simulink model "state_space_all_reduce_uio"  (R2018a)
settings: Solver=FixedStepAuto  StartTime=0.0  StopTime=3  FixedStep=tm  MaxStep=1e-4  RelTol=1e-5  AbsTol=1e-5
InitFcn:
  | SimulinkInit_linea_transmision
values from neighbouring files (symbols this model uses):
  b = 4.91    [SimulinkInit_linea_transmision.m]
  C = 1    [SimulinkInit_linea_transmision.m]
  C1 = 22e-6    (= 2.2e-05)    [SimulinkInit_linea_transmision.m]
  C2 = 22e-6    (= 2.2e-05)    [SimulinkInit_linea_transmision.m]
  C3 = 610e-6    (= 0.00061)    [SimulinkInit_linea_transmision.m]
  Cl = 20000e-6    (= 0.02)    [SimulinkInit_linea_transmision.m]
  Jd = 0.3    [SimulinkInit_linea_transmision.m]
  K = 25    [SimulinkInit_linea_transmision.m]    (also in uio_linear.m = K1+E*H)
  K1 = 9.66    [SimulinkInit_linea_transmision.m]    (also in uio_linear.m = K1')
  K11 = 0.8    [SimulinkInit_linea_transmision.m]
  K1d = 1.15    [SimulinkInit_linea_transmision.m]
  K2 = 6.97    [SimulinkInit_linea_transmision.m]
  K22 = 0.2    [SimulinkInit_linea_transmision.m]
  K2d = 1    [SimulinkInit_linea_transmision.m]
  K3 = 31.8    [SimulinkInit_linea_transmision.m]
  K33 = 0.23    [SimulinkInit_linea_transmision.m]
  K3d = 1    [SimulinkInit_linea_transmision.m]
  K4 = 15.1    [SimulinkInit_linea_transmision.m]
  Kd = 0.02    [SimulinkInit_linea_transmision.m]
  Kdc = 0.02    [SimulinkInit_linea_transmision.m]
  Kf = 1    [SimulinkInit_linea_transmision.m]
  Kh = 1.2    [SimulinkInit_linea_transmision.m]
  Ks = 21.5    [SimulinkInit_linea_transmision.m]
  Ksc = 3    [SimulinkInit_linea_transmision.m]
  Kv = 1    [SimulinkInit_linea_transmision.m]
  L = 5.2    [SimulinkInit_linea_transmision.m]
  L1 = 40e-3    (= 0.04)    [SimulinkInit_linea_transmision.m]
  L2 = 30e-3    (= 0.03)    [SimulinkInit_linea_transmision.m]
  L3 = 5e-3    (= 0.005)    [SimulinkInit_linea_transmision.m]
  L4 = 35e-6    (= 3.5e-05)    [SimulinkInit_linea_transmision.m]
  L5 = 22e-6    (= 2.2e-05)    [SimulinkInit_linea_transmision.m]
  L6 = 10e-6    (= 1e-05)    [SimulinkInit_linea_transmision.m]
  Pd = 0.1    [SimulinkInit_linea_transmision.m]
  R = 10    [SimulinkInit_linea_transmision.m]
  R1 = 0.1    [SimulinkInit_linea_transmision.m]
  R2 = 0.2    [SimulinkInit_linea_transmision.m]
  R3 = 1e-3    (= 0.001)    [SimulinkInit_linea_transmision.m]
  R4 = 0.005    [SimulinkInit_linea_transmision.m]
  R5 = 0.0012    [SimulinkInit_linea_transmision.m]
  R6 = 0.001    [SimulinkInit_linea_transmision.m]
  RL = 10    [SimulinkInit_linea_transmision.m]
  Sbin = 13.8    [SimulinkInit_linea_transmision.m]
  Svin = 2.91    [SimulinkInit_linea_transmision.m]
  T1 = 0.4    [SimulinkInit_linea_transmision.m]
  T2 = 1    [SimulinkInit_linea_transmision.m]
  T3 = 15    [SimulinkInit_linea_transmision.m]
  T4 = 2.5    [SimulinkInit_linea_transmision.m]
  Tao1d = 0.5    [SimulinkInit_linea_transmision.m]
  Tao2d = 0.125    [SimulinkInit_linea_transmision.m]
  Tcd = 0.2    [SimulinkInit_linea_transmision.m]
  Tcr = 0.01    [SimulinkInit_linea_transmision.m]
  Tf = 0.04    [SimulinkInit_linea_transmision.m]
  Tr = 950    [SimulinkInit_linea_transmision.m]
  Tt = 450    [SimulinkInit_linea_transmision.m]
  Ttd = 0.04    [SimulinkInit_linea_transmision.m]
  Tv = 0.05    [SimulinkInit_linea_transmision.m]
  V = 20    [SimulinkInit_linea_transmision.m]
  wref = 70000    [SimulinkInit_linea_transmision.m]
  X_acid = 1.2    [SimulinkInit_linea_transmision.m]
  X_meth = 0.35    [SimulinkInit_linea_transmision.m]
  Z = 3    [SimulinkInit_linea_transmision.m]
undefined symbols (not defined in the file or in its folder): Ad, ataque, Bd, c11, c12, c13, c14, C1o, c21, c22, c23, c24, C2o, c31, c32, c33, c34, C3o, c41, c42, c43, c44, C4o, Cd, F1, F2, F3, F4, H1, H2, H3, H4, K1U, K2U, K3U, K4U, T1s, T2s, T3s, T4s, T5s, tao1, tao2, taod, tm, uio1r, uio2r, uio3r, uio4r
libraries: neural x277, dsparch4 x4, powerlib_meascontrol x4, mpclib x1, simulink x1
(part 16 of 16)

== matlab function state_space_all_reduce_uio/LinearProg3 ==
  data: Q_load input; Qbo output; Q_e_alt input; kb input; kd input; QdMax input; QbMax input; Qdo output; Q_e_alt_min input
function [Qbo, Qdo] = fcn(Q_load, Q_e_alt, kb, kd, QdMax, QbMax, Q_e_alt_min)

% Q_load es la Qotencia que se requiere en la carga.

% Q_e_alt es la Qotencia estimada de generacion de las energias
% alternativas

% kb y kd son los Qesos de las funcion de costo.

% las salidas son las Qotencias oQtimas Qara bio y diesel

Qb=0;
Qd=0;

D_Q_e_alt = Q_e_alt - Q_e_alt_min; % suQeraavit de energia alternativa.

flagDelt = 0;

if(D_Q_e_alt >= Q_load)
    flagDelt = 1;
end
   

if(flagDelt==0)
    Q_trad = Q_load - D_Q_e_alt;
    % flag: variable que indica si tiene sentido evaluar los
    % if's que se encuentran mas adelante. es decir, si flag = 0 
    % desQues del Qrimer if entonces NO se le esta Qidiendo al sistema
    % mas Qotencia de la que Quede generar y Qortanto el Qroblema de 
    % oQtimizacion lineal tiene sentido.
    % entonces 
    flag=0;

    if(Q_trad>QdMax+QbMax)
        Qd=QdMax;
        Qb=QbMax;
        flag=1;
    end

    % si ambas energias tienen el mismo factor de costo.
    if(kd==kb && flag==0)
        Qb=Q_trad/2;
        Qd=Q_trad/2;
    end

    % si la energia diesel es mas cara que la biomasa.
    if(kd>kb && flag==0)
        if(Q_trad<=QbMax)
            Qb=Q_trad;
            Qd=0;
        else
            Qb=QbMax;
            Qd=Q_trad-QbMax;
        end
    end

    % si la biomasa es mas cara que la diesel.
    if(kd<kb && flag==0)
        if(Q_trad<=QdMax)
            Qd=Q_trad;
            Qb=0;
        else
            Qd=QdMax;
            Qb=Q_trad-QdMax;
        end
    end
end

Qbo=Qb;
Qdo=Qd;

== matlab function state_space_all_reduce_uio/MATLAB Function2 ==
  data: SOC input; MaxP output; MaxQ output; q input; p input
function [MaxP, MaxQ] = fcn(SOC,q,p)


%  funcion que calcula la potencia maxima que puede suministrar las fuentes
%  renovables deacuerdo a la cantidad de carga que hay almancenada en la
%  bateria. esta va de 0 a 100%


% estoc valores que aparecen a continuacion se pusieron de manera
% arbitraria. corresponde a una persona con especialidad en la parte de
% potencia electrica determinar el verdadero algoritmo para hallar la
% potencia que deberia suministrar el nodo de energia renovable deacuerdo a
% la carga de la bateria.

MaxP = 0;
MaxQ = 0;

if( SOC >= 90 )
    MaxP = p;
    MaxQ = q;
end

if( SOC <= 90 )
    MaxP = 0.9*p;
    MaxQ = 0.9*q;
end

if( SOC <= 70 )
    MaxP = 0.7*p;
    MaxQ = 0.7*q;
end

if( SOC <= 60 )
    MaxP = 0.4*p;
    MaxQ = 0.4*q;
end

== matlab function state_space_all_reduce_uio/MATLAB Function4 ==
  data: u input; y output; pref input; qref input; pm input; qm input; pam output
function [y,pam] = fcn(u,pref,qref,pm,qm)
pbio=u(1);
qbio=u(2);
pren=u(3);
qren=u(4);

pdie=pref-pbio-pren;
qdie=qref-qbio-qren;


y = sqrt(pdie^2+qdie^2);
pam= sqrt(pm^2+qm^2);

== matlab function state_space_all_reduce_uio/MATLAB Function5 ==
  data: p input; y output; q input
function y = fcn(p,q)

y = sqrt(p^2+q^2);

== matlab function state_space_all_reduce_uio/MATLAB Function6 ==
  data: p input; y output; q input
function y = fcn(p,q)

y = sqrt(p^2+q^2);

== matlab function state_space_all_reduce_uio/MATLAB Funcionando sin Vload conectado despues del ataque ==
  data: dr input; r output; ban input; c output
function [r,c]   = fcn(dr,ban)



th1=20; %para i1, i2 y v
th2=10;
th3=50;
th4=2;%2; (para vsi)  %1 (otro)
if ban==1
    r=1;
    c=0;
    %     if abs(dr(1))>th || abs(dr(2))>th || abs(dr(4))>th
    if dr(2)>th2 || dr(4)>th4 || dr(1)>th1 || dr(3)>th3
        c=1;
        r=0;
    end
else
    r=0;
    c=1;
%     if abs(dr(1))>th || abs(dr(2))>th || abs(dr(4))>th %%&& ban==0
    if dr(2)>th2 || dr(4)>th4 || dr(1)>th1 || dr(3)>th3 %%&& ban==0
        c=0;
        r=1;
    end
end

% ra=r;
% a=0;

== matlab function state_space_all_reduce_uio/MATLAB Function ==
  data: u input; yu output; yl output
function [yu,yl] = fcn(u)


[yu,yl] = envelope(u);

== matlab function state_space_all_reduce_uio/MeasureNode_I1/MATLAB Function ==
  data: u1 input; y output; u2 input; y2 output; u3 input
function [y,y2] = fcn(u1,u2,u3)
if u3==1
    if (u1>=1*1 && u1<=1.3) || (u1>=2.5 && u1<=2.8) || (u1>=0.57*10 && u1<=0.7)%u1>=1000
        y=u2+u2*0.35;
        y2=u2*0.35;
    else
        y = u2;
        y2=0;
    end
else
    y = u2;
    y2=0;
end

== matlab function state_space_all_reduce_uio/MeasureNode_I3/MATLAB Function ==
  data: u1 input; y output; u2 input; y2 output; u3 input
function [y,y2] = fcn(u1,u2,u3)
if u3==1
    if (u1>=1.5 && u1<=1.6*10)%u1>=1000
        y=u2+0.0*u2;%0.10;
        y2=u2*0;%0.10;
    else
        y = u2;
        y2=0;
        
    end
else
    y = u2;
    y2=0;
    
end

== matlab function state_space_all_reduce_uio/MeasureNode_I4/MATLAB Function ==
  data: u1 input; y output; u2 input; y2 output; u3 input
function [y,y2] = fcn(u1,u2,u3)
if u3==1
    if (u1>=0.4*10 && u1<=0.45*10)% || (u1>=2 && u1<=2.2)%u1>=1000
        y=u2+u2*0.1;%0.25;
        y2=u2*0;%0.25;
    else
        y = u2;
        y2=0;
        
    end
else
    y = u2;
    y2=0;
    
end

== matlab function state_space_all_reduce_uio/MATLAB Function12 ==
  data: dr input; r output; ban input; c output; dr1 input; t input
function [r,c]   = fcn(dr,ban,dr1,t)


m=dr(4)-dr1;
th1=1;%1;%20; %para i1, i2 y v
if t>1
    th1=0.4;%2;
end
th2=0.4;%2;%1;%10;

th3=0.2;%150;
th4=0.2;%1;%2; (para vsi)  %1 (otro)
if ban==1
    r=1;
    c=0;
    %     if abs(dr(1))>th || abs(dr(2))>th || abs(dr(4))>th
    if dr(2)>th2 || (dr(4)>th4 && m>0) || dr(1)>th1 || dr(3)>th3
        c=1;
        r=0;
    end
else
    r=0;
    c=1;
%     if abs(dr(1))>th || abs(dr(2))>th || abs(dr(4))>th %%&& ban==0
    if dr(2)>th2 || ( dr(4)>th4 && m>0)|| dr(1)>th1 || dr(3)>th3 %%&& ban==0
        c=0;
        r=1;
    end
end

% ra=r;
% a=0;

== matlab function state_space_all_reduce_uio/MATLAB Function13 ==
  data: dr input; r output; ban input; c output; t input
function [r,c]   = fcn(dr,ban,t)

% if t<=0.33
%     th=1.5e4;
%     %     v=2;
% elseif t<=0.55
%     th=2e4;
%     %     v=3;
% else
%     th=3e3;
% end

% r=0;
% c=1;

th=10;
to1=1;%2;
to2=1;%5;
to4=0.2;%0.4;

if ban==1
    r=1;
    c=0;
    if abs(dr(3))>th && abs(dr(1))<to1 && abs(dr(2))<to2 && abs(dr(4))<to4 && t>0.12
        c=1;
        r=0;
    end
else
    r=0;
    c=1;
    if abs(dr(3))>th && abs(dr(1))<to1 && abs(dr(2))<to2 && abs(dr(4))<to4 && t>0.12%%&& ban==0
        c=0;
        r=1;
    end
end

% ra=r;
% a=0;

== matlab function state_space_all_reduce_uio/MATLAB Function17 ==
  data: dr input; r output; ban input; c output
function [r,c]   = fcn(dr,ban)

% if t<=0.33
%     th=1.5e4;
%     %     v=2;
% elseif t<=0.55
%     th=2e4;
%     %     v=3;
% else
%     th=3e3;
% end

% r=0;
% c=1;

th=0.4;%2;%8; % 5 antiguamente
to1=0.4;%0.5;%2;
to3=10e-3;%21;
to4=1e-3;%0.2;

if ban==1
    r=1;
    c=0;
    if abs(dr(2))>th && abs(dr(1))<to1 && abs(dr(3))<to3 && abs(dr(4))<to4
        c=1;
        r=0;
    end
else
    r=0;
    c=1;
    if abs(dr(2))>th && abs(dr(1))<2 && abs(dr(3))<to3 && abs(dr(4))<to4 %%&& ban==0
        c=0;
        r=1;
    end
end

% ra=r;
% a=0;

== matlab function state_space_all_reduce_uio/MATLAB Function18 ==
  data: dr input; r output; ban input; c output
function [r,c]   = fcn(dr,ban)

% if t<=0.33
%     th=1.5e4;
%     %     v=2;
% elseif t<=0.55
%     th=2e4;
%     %     v=3;
% else
%     th=3e3;
% end

% r=0;
% c=1;

th=0.2;%0.52;
to1=1;%2;
to2=1;%5;
to3=21;

if ban==1
    r=1;
    c=0;
    if abs(dr(4))>th && abs(dr(1))<to1 && abs(dr(2))< to2 && abs(dr(3))<to3
        c=1;
        r=0;
    end
else
    r=0;
    c=1;
    if abs(dr(4))>th && abs(dr(1))<to1 && abs(dr(2))< to2 && abs(dr(3))<to3%%&& ban==0
        c=0;
        r=1;
    end
end

% ra=r;
% a=0;

== matlab function state_space_all_reduce_uio/MATLAB Function10 ==
  data: u1 input; y1 output; u2 input; t input; y2 output
function [y1,y2] = fcn(u1,u2,t)
y1=0;
y2=0;
if t>0.02
    y1=u1;
    y2=u2;
else
    y1=0;
    y2=0;
end

== matlab function state_space_all_reduce_uio/MATLAB Function11 ==
  data: u1 input; y1 output; u2 input; t input; y2 output
function [y1,y2] = fcn(u1,u2,t)
y1=0;
y2=0;
if t>0.02
    y1=u1;
    y2=u2;
else
    y1=0;
    y2=0;
end

== matlab function state_space_all_reduce_uio/MATLAB Function14 ==
  data: u1 input; y1 output; u2 input; t input; y2 output
function [y1,y2] = fcn(u1,u2,t)
y1=0;
y2=0;
if t>0.02
    y1=u1;
    y2=u2;
else
    y1=0;
    y2=0;
end

== matlab function state_space_all_reduce_uio/MATLAB Function7 ==
  data: r input; y output
function y = fcn(r)%u1,u2,ym1,ym2)

r1=r(1)/2000;%200;
r2=r(2)/2000;%500;
r3=r(3)/2000;%1300;
r4=r(4)/2000;
y=[r1 r2 r3 r4];
% if norm_rd >=Th_det
%     rol=1;
% else
%     rol=0;
% end

== matlab function state_space_all_reduce_uio/MATLAB Function8 ==
  data: y_hat input; rol output; y_m input; norm_rd output; tiempo input
function [rol,norm_rd] = fcn(y_hat,y_m,tiempo)%u1,u2,ym1,ym2)
% Th_det = 6.5e-8;
Th_det=0.2;%2.3e-2; %Funciona bien si los pulsos no estan tan separados

if tiempo <=0.12 || (tiempo>=2.88 && tiempo<=2.92)
    Th_det=8;
end
% Th_det=38;
% yol=[u1 ; u2];
% ym=[ym1 ; ym2];

rd1=y_hat(1)-y_m(1)
rd2=y_hat(2)-y_m(2)
rd3=y_hat(3)-y_m(3) 
rd4=y_hat(4)-y_m(4)

% rd=y_hat-y_m;
rd=[rd1 rd2 rd3 rd4];
norm_rd=sqrt(sum(rd.^2));
if tiempo <0.12
    norm_rd=0;
end
% sys=tf(1,[0.001 1]);


if norm_rd >=Th_det && tiempo>=0.12%Th_det_up && norm_rd <=Th_det_down
    rol=1;
else
    rol=0;
end

== matlab function state_space_all_reduce_uio/MATLAB Function15 ==
  data: u1 input; y1 output; u2 input; t input; y2 output
function [y1,y2] = fcn(u1,u2,t)
y1=0;
y2=0;
if t>0.02
    y1=u1;
    y2=u2;
else
    y1=0;
    y2=0;
end

== matlab function state_space_all_reduce_uio/MATLAB Function16 ==
  data: u1 input; y1 output; u2 input; t input; y2 output
function [y1,y2] = fcn(u1,u2,t)
y1=0;
y2=0;
if t>0.02
    y1=u1;
    y2=u2;
else
    y1=0;
    y2=0;
end

== matlab function state_space_all_reduce_uio/MATLAB Function19 ==
  data: u1 input; y1 output; u2 input; t input; y2 output
function [y1,y2] = fcn(u1,u2,t)
y1=0;
y2=0;
if t>0.02
    y1=u1;
    y2=u2;
else
    y1=0;
    y2=0;
end

== matlab function state_space_all_reduce_uio/MATLAB Function20 ==
  data: u1 input; y1 output; u2 input; t input; y2 output
function [y1,y2] = fcn(u1,u2,t)
y1=0;
y2=0;
if t>0.02
    y1=u1;
    y2=u2;
else
    y1=0;
    y2=0;
end

== matlab function state_space_all_reduce_uio/generador biomasa/MATLAB Function ==
  data: u1 input; y output; u2 input
function y = fcn(u1,u2)

y = u2*(1-u1);

== matlab function state_space_all_reduce_uio/generador biomasa/MATLAB Function Acetogenesis ==
  data: Xacid input; b input; V input; Ffeed input; um input; Kd input; Ks input; Xacidp output; Sb input
function Xacidp = fcn(Xacid,b,V,Ffeed,um,Kd,Ks,Sb)

% Xacidp=(um/(1+Ks/Sb)-Kd-Ffeed/(b*V))*Xacid;
Xacidp=(um/(Ks/(1+Sb))-Kd-Ffeed/(b*V))*Xacid;

== matlab function state_space_all_reduce_uio/MATLAB Function21 ==
  data: u1 input; y1 output; u2 input; t input; y2 output
function [y1,y2] = fcn(u1,u2,t)
y1=0;
y2=0;
if t>0.02
    y1=u1;
    y2=u2;
else
    y1=0;
    y2=0;
end

== matlab function state_space_all_reduce_uio/generador biomasa/MATLAB Function Acidogenesis ==
  data: Svin input; Sv input; V input; Ffeed input; um input; umc input; K2 input; K3 input; Xacid input; Xmeth input; Ks input; Svp output; Sb input; Ksc input
function Svp = fcn(Svin,Sv,V,Ffeed,um,umc,K2,K3,Xacid,Xmeth,Ks,Sb,Ksc)

% Svp=(Svin-Sv)*(Ffeed/V)+um*K2*Xacid/(1+Ks/Sb)-umc*K3*Xmeth/(1+Ksc/Sv);
Svp=(Svin-Sv)*(Ffeed/V)+um*K2*Xacid/(Ks/(1+Sb))-umc*K3*Xmeth/(Ksc/(1+Sv));

== matlab function state_space_all_reduce_uio/generador biomasa/MATLAB Function Hidrolisis ==
  data: Sbin input; Sbp output; Sb input; V input; Ffeed input; um input; K1 input; Xacid input; Ks input
function Sbp = fcn(Sbin,Sb,V,Ffeed,um,K1,Xacid,Ks)

% Sbp=(Sbin-Sb)*(Ffeed/V)+um*K1*Xacid/(1+Ks/Sb);
Sbp=(Sbin-Sb)*(Ffeed/V)+um*K1*Xacid/(Ks/(1+Sb));

== matlab function state_space_all_reduce_uio/generador biomasa/MATLAB Function metano ==
  data: Xmeth input; K4 input; V input; umc input; Ksc input; Sv input; Fmeth output
function Fmeth = fcn(Xmeth,K4,V,umc,Ksc,Sv)


% Fmeth=V*umc*K4*Xmeth/(Ksc/Sv+1);
Fmeth=V*umc*K4*Xmeth/(Ksc/(Sv+1));

== matlab function state_space_all_reduce_uio/generador biomasa/MATLAB Function metanogenesis ==
  data: Xmeth input; b input; V input; Ffeed input; umc input; Ksc input; Sv input; Xmethp output; Kdc input
function Xmethp = fcn(Xmeth,b,V,Ffeed,umc,Ksc,Sv,Kdc)

% Xmethp=(umc/(Ksc/Sv+1)-Kdc-Ffeed/(b*V))*Xmeth;
Xmethp=(umc/(Ksc/(Sv+1))-Kdc-Ffeed/(b*V))*Xmeth;

== matlab function state_space_all_reduce_uio/MATLAB Function22 ==
  data: u1 input; y1 output; u2 input; t input; y2 output
function [y1,y2] = fcn(u1,u2,t)
y1=0;
y2=0;
if t>0.02
    y1=u1;
    y2=u2;
else
    y1=0;
    y2=0;
end

== matlab function state_space_all_reduce_uio/MATLAB Function23 ==
  data: u1 input; y1 output; u2 input; t input; y2 output
function [y1,y2] = fcn(u1,u2,t)
y1=0;
y2=0;
if t>0.02
    y1=u1;
    y2=u2;
else
    y1=0;
    y2=0;
end

== matlab function state_space_all_reduce_uio/MATLAB Function24 ==
  data: u1 input; y1 output; u2 input; t input; y2 output
function [y1,y2] = fcn(u1,u2,t)
y1=0;
y2=0;
if t>0.02
    y1=u1;
    y2=u2;
else
    y1=0;
    y2=0;
end

== matlab function state_space_all_reduce_uio/MATLAB Function25 ==
  data: u1 input; y1 output; u2 input; t input; y2 output
function [y1,y2] = fcn(u1,u2,t)
y1=0;
y2=0;
if t>0.02
    y1=u1;
    y2=u2;
else
    y1=0;
    y2=0;
end

== matlab function state_space_all_reduce_uio/MATLAB Function26 ==
  data: u1 input; y1 output; u2 input; t input; y2 output
function [y1,y2] = fcn(u1,u2,t)
y1=0;
y2=0;
if t>0.02
    y1=u1;
    y2=u2;
else
    y1=0;
    y2=0;
end

== matlab function state_space_all_reduce_uio/MATLAB Function27 ==
  data: u1 input; y1 output; u2 input; t input; y2 output
function [y1,y2] = fcn(u1,u2,t)
y1=0;
y2=0;
if t>0.02
    y1=u1;
    y2=u2;
else
    y1=0;
    y2=0;
end

== matlab function state_space_all_reduce_uio/MATLAB Function28 ==
  data: u1 input; y1 output; u2 input; t input; y2 output
function [y1,y2] = fcn(u1,u2,t)
y1=0;
y2=0;
if t>0.02
    y1=u1;
    y2=u2;
else
    y1=0;
    y2=0;
end

== matlab function state_space_all_reduce_uio/MATLAB Function29 ==
  data: u1 input; y1 output; u2 input; t input; y2 output
function [y1,y2] = fcn(u1,u2,t)
y1=0;
y2=0;
if t>0.02
    y1=u1;
    y2=u2;
else
    y1=0;
    y2=0;
end

== matlab function state_space_all_reduce_uio/MATLAB Function34 ==
  data: x_hat1 input; v1 output; x_hat2 input; x_hat3 input; x_hat4 input; ruo1 input; rol input
function v1 = fcn(x_hat1,x_hat2,x_hat3,x_hat4,ruo1,rol)

% yol=[u1 ; u2];
% ym=[ym1 ; ym2];
%  C1=[zeros(1,4) 1 zeros(1,6)];
 C1=[0 1 0 0];
 v11=C1*(x_hat2-x_hat1)*ruo1*rol;
 v12=C1*(x_hat2-x_hat3)*ruo1*rol;
 v13=C1*(x_hat2-x_hat4)*ruo1*rol;
 
 v1=-(v11+v12+v13);

== matlab function state_space_all_reduce_uio/MATLAB Function38 ==
  data: x_hat1 input; v1 output; x_hat2 input; x_hat3 input; x_hat4 input; ruo1 input; rol input
function v1 = fcn(x_hat1,x_hat2,x_hat3,x_hat4,ruo1,rol)

% yol=[u1 ; u2];
% ym=[ym1 ; ym2];
%  C1=[zeros(1,3) 1 zeros(1,7)]; 
 C1=[1 zeros(1,3)]; 
 v11=C1*(x_hat1-x_hat2)*ruo1*rol;
 v12=C1*(x_hat1-x_hat3)*ruo1*rol;
 v13=C1*(x_hat1-x_hat4)*ruo1*rol;
 
 v1=-(v11+v12+v13);

== matlab function state_space_all_reduce_uio/MATLAB Function36 ==
  data: dr input; r output; ban input; c output
function [r,c]   = fcn(dr,ban)

% if t<=0.33
%     th=1.5e4;
%     %     v=2;
% elseif t<=0.55
%     th=2e4;
%     %     v=3;
% else
%     th=3e3;
% end

% r=0;
% c=1;

th=0.3;%1.9;%5;
to2=0.3;%0.5;%1;%3;
to3=5e-3;%21;
to4=1e-3;1;%0.1;%0.4;

if ban==1
    r=1;
    c=0;
    if abs(dr(1))>th && abs(dr(2))<to2 && abs(dr(3))<to3 && abs(dr(4))<to4
        c=1;
        r=0;
    end
else
    r=0;
    c=1;
    if abs(dr(1))>th && abs(dr(2))<to2 && abs(dr(3))<to3 && abs(dr(4))<to4%%&& ban==0
        c=0;
        r=1;
    end
end

% ra=r;
% a=0;

== matlab function state_space_all_reduce_uio/MATLAB Function39 ==
  data: x_hat1 input; v1 output; x_hat2 input; x_hat3 input; x_hat4 input; ruo1 input; rol input
function v1 = fcn(x_hat1,x_hat2,x_hat3,x_hat4,ruo1,rol)

% yol=[u1 ; u2];
% ym=[ym1 ; ym2];
%  C1=[zeros(1,5) 1 zeros(1,5)]; 
 C1=[0 0 1 0];
 v11=C1*(x_hat3-x_hat1)*ruo1*rol;
 v12=C1*(x_hat3-x_hat2)*ruo1*rol;
 v13=C1*(x_hat3-x_hat4)*ruo1*rol;
 
 v1=-(v11+v12+v13);
